simulink model "pid_simulacao"  (R2014a)
settings: Solver=ode3  StartTime=0.0  StopTime=100  FixedStep=0.1  RelTol=1e-3
settings Model: Creator=icaro  LastModifiedBy=Aluno IC

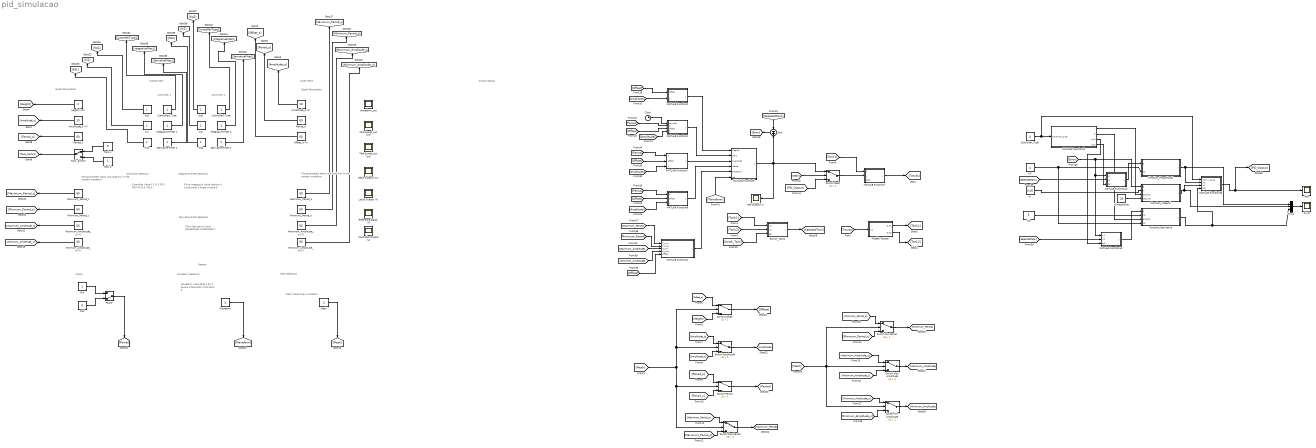
== system pid_simulacao ==
  note: Output Signals
  note: Controller
      | Value
      |
      | P
      | 1
      |
      | PI
      | 2
      |
      | PD
      | 3
      |
      | PID
      | 4
      |
      | PI-D
      | 5
      |
      | I-PD
      | 6
  note: Controller Selection
  note: Signal Parameters
  note: Mesh
      | Value
      |
      | Open
      | 1
      |
      | Closed
      | 2
  note: Mesh Selection
  note: Power
  note: Waveform
      | Value
      |
      | Step
      | 1
      |
      | Sin
      | 2
      |
      | Square
      | 3
      |
      | Sawtooth
      | 4
      |
      | Ramdom
      | 5
  note: Waveform Selection
  note: General
  note: Controller 1
  note: The parameters below are used only in the random waveform
  note: Signal Parameters
  note: The parameters below are used only in the random waveform
  note: Open Mesh
  note: Controller 2
  note: Filtro Derivativo
      | Value
      |
      | Desabilitado
      | 0
      |
      | Habilitado
      | 1
  note: Filtro Integrativo
      | Value
      |
      | Nenhum
      | 0
      |
      | Condicional
      | 1
      |
      | Reset windup
      | 6
  note: Integrative Filter Selection
  note: Derivative Filter Selection
  note: Closed Mesh
  Amplitude_c (V) : Constant  Value=10
  Amplitude_o (V) : Constant  Value=10
  Clock : Clock
  Controller Output (V) : Scope
      settings: TimeRange=10  YMin=2.5  YMax=10  SaveName=meshoutput4
  Controller1 Type : Constant
  Controller2 Type : Constant
  Controller_Type : Constant  Value=4
  Derivative Filter 1 : Constant
  Derivative Filter 2 : Constant
  Function_Derivative : MATLAB Function  TreatAsAtomicUnit=on
  Function_Integral : MATLAB Function  TreatAsAtomicUnit=on
  Function_Proportional : MATLAB Function  TreatAsAtomicUnit=on
  Height (cm) : Constant  Value=2
  Integrative Filter 1 : Constant
  Integrative Filter 2 : Constant
  KD : Constant  Value=5
  KI : Constant  Value=0.05
  KP : Constant  Value=4
  Kd1 : Constant
  Kd2 : Constant
  Ki1 : Constant
  Ki2 : Constant
  Kp1 : Constant
  Kp2 : Constant
  Locks Output (V) : Scope
      settings: TimeRange=10  YMin=2.5  YMax=10  SaveName=meshoutput2
  MATLAB Function1 : MATLAB Function  TreatAsAtomicUnit=on
  MATLAB Function11 : MATLAB Function  TreatAsAtomicUnit=on
  MATLAB Function13 : MATLAB Function  TreatAsAtomicUnit=on
  MATLAB Function14 : MATLAB Function  TreatAsAtomicUnit=on
  MATLAB Function16 : MATLAB Function  TreatAsAtomicUnit=on
  MATLAB Function2 : MATLAB Function  TreatAsAtomicUnit=on
  MATLAB Function3 : MATLAB Function  TreatAsAtomicUnit=on
  MATLAB Function4 : MATLAB Function  TreatAsAtomicUnit=on
  MATLAB Function5 : MATLAB Function  TreatAsAtomicUnit=on
  MATLAB Function6 : MATLAB Function  TreatAsAtomicUnit=on
  MATLAB Function7 : MATLAB Function  TreatAsAtomicUnit=on
  Maximum_Amplitude_c (V) : Constant  Value=60
  Maximum_Amplitude_o (V) : Constant  Value=60
  Maximum_Period_c : Constant  Value=60
  Maximum_Period_o : Constant  Value=60
  Mesh : Constant  Value=2
  Mesh Output (V)1 : Scope
      settings: TimeRange=10  YMin=2.5  YMax=10  SaveName=meshoutput1
  Minimum_Amplitude_c (V) : Constant  Value=60
  Minimum_Amplitude_o (V) : Constant  Value=60
  Minimum_Period_c : Constant  Value=60
  Minimum_Period_o : Constant  Value=60
  Modelo Tanque : Subsystem
  Mux2 : Mux  Inputs=3
  OFF : Constant  Value=0
  ON : Constant
  Offset_o (V) : Constant  Value=60
  P-I-D : Scope
      settings: ShowLegends=on  TimeRange=300  YMin=-100  YMax=100  SaveName=PID
  PID : Scope
      settings: TimeRange=100  YMin=0  YMax=100
  Period_c : Constant  Value=60
  Period_o : Constant  Value=60
  Power : ManualSwitch  CurrentSetting=0
  Ref Output (V) : Scope
      settings: TimeRange=100  SaveName=muxoutput
  Reference Signal (V) : Scope
      settings: TimeRange=10  YMin=2.5  YMax=10  SaveName=meshoutput3
  Sum : Sum  Inputs=-+
  Switch Amplitude : Switch  Criteria=u2 > Threshold  Threshold=1
  Switch Max Amplitude : Switch  Criteria=u2 > Threshold  Threshold=1
  Switch Max Period : Switch  Criteria=u2 > Threshold  Threshold=1
  Switch Mesh : Switch  Criteria=u2 > Threshold  Threshold=1
  Switch Min Amplitude : Switch  Criteria=u2 > Threshold  Threshold=1
  Switch Min Period : Switch  Criteria=u2 > Threshold  Threshold=1
  Switch Offset : Switch  Criteria=u2 > Threshold  Threshold=1
  Switch Period : Switch  Criteria=u2 > Threshold  Threshold=1
  Switch_Tanks : MATLAB Function  TreatAsAtomicUnit=on
  Tank 1 : Constant  Value=0
  Tank 2 : Constant
  Tank1Level_out (cm) : Scope
      settings: TimeRange=10  YMin=4.125  YMax=4.5  SaveName=muxoutput2
  Tank2Level_out (cm) : Scope
      settings: TimeRange=10  YMin=4.125  YMax=4.5  SaveName=muxoutput3
  Tank_Switch : ManualSwitch
  Waveform : Constant  Value=3
  Waveform_out : Scope
      settings: TimeRange=10  YMin=4.125  YMax=4.5  SaveName=muxoutput1
  WindupValue : Constant  Value=20
  wires:
  Clock/1 -> MATLAB Function1/1(counter)
  MATLAB Function7/1(y) -> [Travas]
  MATLAB Function5/1(y) -> Switch Mesh/1, Ref Output (V)/1, Sum/2
  Switch Mesh/1 -> MATLAB Function7/2(u)
  ON/1 -> Power/1
  OFF/1 -> Power/2
  Tank 1/1 -> Tank_Switch/1
  Tank 2/1 -> Tank_Switch/2
  Function_Proportional/1(y) -> MATLAB Function16/2(pro), Mux2/1
  Function_Integral/1(y) -> MATLAB Function16/3(int), Mux2/2
  Sum/1 -> [Error]
  MATLAB Function11/1(i) -> Function_Integral/3(enable)
  KP/1 -> Function_Derivative/4(Kp), Function_Proportional/2(Kp)
  MATLAB Function11/2(d) -> Function_Derivative/3(enable)
  Controller_Type/1 -> MATLAB Function16/1(control_type), MATLAB Function11/1(controller_type)
  MATLAB Function16/1(y) -> [PID_Output], PID/1
  Mux2/1 -> P-I-D/1
  MATLAB Function13/1(y) -> Function_Derivative/1(e)
  MATLAB Function11/3(swd) -> MATLAB Function13/3(sel)
  MATLAB Function14/1(y) -> Function_Proportional/1(e)
  MATLAB Function11/4(swp) -> MATLAB Function14/3(sel)
  KI/1 -> Function_Integral/2(Ki)
  WindupValue/1 -> Function_Integral/4(sat_max)
  KD/1 -> Function_Derivative/2(Kd)
  Function_Derivative/1(y) -> MATLAB Function16/4(der), Mux2/3
  [Travas] -> Modelo Tanque/1(In1)
  Modelo Tanque/1(Out1) -> [Tank1]
  Modelo Tanque/2(Out2) -> [Tank2]
  [Tank1] -> MATLAB Function7/1(h)
  Height (cm)/1 -> [Height]
  Tank_Switch/1 -> [Tank_Switch]
  Amplitude_c (V)/1 -> [Amplitude_c]
  Period_c/1 -> [Period_c]
  Maximum_Period_c/1 -> [Maximum_Period_c]
  Minimum_Period_c/1 -> [Minimum_Period_c]
  Maximum_Amplitude_c (V)/1 -> [Maximum_Amplitude_c]
  Minimum_Amplitude_c (V)/1 -> [Minimum_Amplitude_c]
  Waveform/1 -> [Waveform]
  Mesh/1 -> [Mesh]
  Power/1 -> [Power]
  Amplitude_o (V)/1 -> [Amplitude_o]
  Period_o/1 -> [Period_o]
  Offset_o (V)/1 -> [Offset_o]
  Maximum_Period_o/1 -> [Maximum_Period_o]
  Minimum_Period_o/1 -> [Minimum_Period_o]
  Maximum_Amplitude_o (V)/1 -> [Maximum_Amplitude_o]
  Minimum_Amplitude_o (V)/1 -> [Minimum_Amplitude_o]
  [Mesh] -> Switch Max Period/2, Switch Period/2, Switch Offset/2, Switch Amplitude/2
  [Height] -> Switch Offset/3
  [Offset_o] -> Switch Offset/1
  [Amplitude_o] -> Switch Amplitude/1
  [Amplitude_c] -> Switch Amplitude/3
  [Period_c] -> Switch Period/3
  [Period_o] -> Switch Period/1
  [Maximum_Period_c] -> Switch Max Period/3
  [Maximum_Period_o] -> Switch Max Period/1
  [Minimum_Period_c] -> Switch Min Period/3
  [Minimum_Period_o] -> Switch Min Period/1
  [Maximum_Amplitude_c] -> Switch Max Amplitude/3
  [Maximum_Amplitude_o] -> Switch Max Amplitude/1
  [Minimum_Amplitude_o] -> Switch Min Amplitude/1
  [Minimum_Amplitude_c] -> Switch Min Amplitude/3
  Switch Offset/1 -> [Offset]
  Switch Amplitude/1 -> [Amplitude]
  Switch Period/1 -> [Period]
  Switch Max Period/1 -> [Maximum_Period]
  Switch Min Period/1 -> [Minimum_Period]
  Switch Min Amplitude/1 -> [Minimum_Amplitude]
  Switch Max Amplitude/1 -> [Maximum_Amplitude]
  [Offset] -> MATLAB Function2/1(offset)
  [Amplitude] -> MATLAB Function2/2(A)
  [Amplitude] -> MATLAB Function1/4(A)
  [Offset] -> MATLAB Function1/3(offset)
  [Period] -> MATLAB Function1/2(T)
  [Amplitude] -> MATLAB Function6/3(A)
  [Offset] -> MATLAB Function6/2(offset)
  [Period] -> MATLAB Function6/1(T)
  [SelectedTank] -> MATLAB Function13/2(x2)
  [SelectedTank] -> MATLAB Function14/2(x2)
  [Tank2] -> Switch_Tanks/2(x2)
  [Tank1] -> Switch_Tanks/1(x1)
  Switch_Tanks/1(y) -> [SelectedTank]
  [Switch_Tank] -> Switch_Tanks/3(sel)
  [Offset] -> MATLAB Function3/2(offset)
  [Period] -> MATLAB Function3/1(T)
  [Amplitude] -> MATLAB Function3/3(A)
  [Maximum_Period] -> MATLAB Function4/1(T_min)
  [Minimum_Period] -> MATLAB Function4/2(T_max)
  [Maximum_Amplitude] -> MATLAB Function4/3(A_min)
  [Minimum_Amplitude] -> MATLAB Function4/4(A_max)
  [Offset] -> MATLAB Function4/5(offset)
  MATLAB Function4/1(y) -> MATLAB Function5/5(aleatoria)
  [Waveform] -> MATLAB Function5/6(sel)
  MATLAB Function6/1(y) -> MATLAB Function5/4(dente)
  MATLAB Function3/1(y) -> MATLAB Function5/3(quadrada)
  MATLAB Function1/1(y) -> MATLAB Function5/2(seno)
  MATLAB Function2/1(y) -> MATLAB Function5/1(degrau)
  [Error] -> MATLAB Function14/1(x1), MATLAB Function13/1(x1), Function_Integral/1(e)
  [SelectedTank] -> Sum/1
  [PID_Output] -> Switch Mesh/3
  [Mesh] -> Switch Mesh/2
  [Mesh] -> Switch Min Amplitude/2, Switch Max Amplitude/2, Switch Min Period/2
  Kp1/1 -> [Kp1]
  Ki1/1 -> [Ki1]
  Kd1/1 -> [Kd1]
  Controller1 Type/1 -> [ControllerType1]
  Integrative Filter 1/1 -> [IntegrativeFilter1]
  Derivative Filter 1/1 -> [DerivativeFilter1]
  Kp2/1 -> [Kp2]
  Ki2/1 -> [Ki2]
  Kd2/1 -> [Kd2]
  Derivative Filter 2/1 -> [DerivativeFilter2]
  Integrative Filter 2/1 -> [IntegrativeFilter2]
  Controller2 Type/1 -> [ControllerType2]

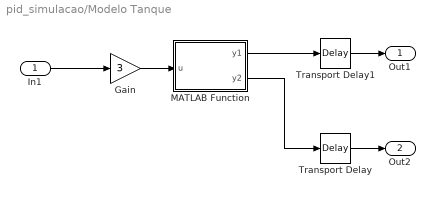
== system pid_simulacao/Modelo Tanque ==
  In1 : Inport
  Gain : Gain  Gain=3
  MATLAB Function : MATLAB Function  TreatAsAtomicUnit=on
  Transport Delay : TransportDelay  DelayTime=2
  Transport Delay1 : TransportDelay  DelayTime=2
  Out1 : Outport
  Out2 : Outport  Port=2
  wires:
  Gain/1 -> MATLAB Function/1(u)
  Transport Delay/1 -> Out2/1
  Transport Delay1/1 -> Out1/1
  MATLAB Function/1(y1) -> Transport Delay1/1
  MATLAB Function/2(y2) -> Transport Delay/1
  In1/1 -> Gain/1

== matlab function pid_simulacao/Modelo Tanque/MATLAB Function ==
  data: u input; y1 output; y2 output
function [y1, y2]= fcn(u)

persistent A1
persistent A2
persistent a1
persistent a2
persistent km
persistent g
persistent t
persistent h1
persistent h2

if(isempty(t))
    A1 = pi*(4.445/2)^2;           %Area transversal do tanque 1
    A2 = pi*(4.445/2)^2;           %Area transversal do tanque 2
    a1 = (0.445/2)^2*pi;     %Area transversal da tubulação de saida em t1 
    a2 =(0.445/2)^2*pi;    %Area transversal da tubulação de saida em t2
    km = 3.3;                %Constante do Motor
    g  = 980.665;               %Constante da gravidade
    h1 = 0;
    h2 = 0;
    t = 10^-1;
end

dh1 = ((km*u) - a1*sqrt(2*g*h1))/A1;
h1 = h1 + t*dh1;
if(h1<0)
    h1 = 0;
end
dh2 = (a1*sqrt(2*g*h1) - a2*sqrt(2*g*h2))/A2;
h2 = h2 + t*dh2;
if(h2<0)
    h2 = 0;
end

y1 = h1;
y2 = h2;

end

== matlab function pid_simulacao/MATLAB Function1 ==
  data: counter input; y output; T input; offset input; A input
function y = seno(counter, T, offset, A)

%counter = cast(counter, 'double');

y = A*sin(counter*2*pi/T) + offset;

== matlab function pid_simulacao/MATLAB Function2 ==
  data: offset input; y output; A input
function y = degrau(offset, A)



y = A + offset;

== matlab function pid_simulacao/MATLAB Function3 ==
  data: y output; T input; offset input; A input
function y = quadrada(T, offset, A)

persistent counter_q;

if isempty(counter_q)
   counter_q = 0; 
end

counter_q = counter_q + 1;

if (counter_q <= 5*T)
    y = -A + offset;
elseif (counter_q > 5*T)
    y = A + offset;
else
    y = 0;
end

if (counter_q >= 10*T)
   counter_q = 0; 
end

== matlab function pid_simulacao/MATLAB Function4 ==
  data: T_min input; y output; T_max input; A_min input; A_max input; offset input
function y = aleatoria(T_min, T_max, A_min, A_max, offset)

persistent T_now;
persistent A_now;
persistent counter_a;

if isempty(counter_a)
    T_now = T_min + (T_max - T_min)*rand;
    A_now = A_min + (A_max - A_min)*rand + offset;
    counter_a = 0;
end

counter_a = counter_a + 1;

y = A_now;

if (counter_a >= T_now*10)
    T_now = T_min + (T_max - T_min)*rand;
    A_now = A_min + (A_max - A_min)*rand + offset;
    counter_a = 0;
end

== matlab function pid_simulacao/MATLAB Function5 ==
  data: degrau input; y output; seno input; quadrada input; dente input; aleatoria input; sel input
function y = mux(degrau, seno, quadrada, dente, aleatoria, sel)

switch sel
    case 1
        y = degrau;
    case 2
        y = seno;
    case 3
        y = quadrada;
    case 4
        y = dente;
    case 5
        y = aleatoria;
    otherwise
        y = 0;
end

== matlab function pid_simulacao/MATLAB Function6 ==
  data: y output; T input; offset input; A input
function y = dente(T, offset, A)

persistent counter_d;

if isempty(counter_d)
   counter_d = 0; 
end


y = counter_d*A*2/(10*T) + offset - A;

counter_d = counter_d + 1;

if (counter_d > T*10)
   counter_d = 0;
end

== matlab function pid_simulacao/Function_Proportional ==
  data: e input; y output; Kp input
function y = proportional(e, Kp)

y = Kp*e;

== matlab function pid_simulacao/MATLAB Function7 ==
  data: h input; u input; y output; start input
    function y = travas(h, u, start)
%#codegen
h_max = 30;

%Trava de tensÃ£o
if(u < -4)
    u = -4;
end
if(u > 4)
    u = 4;
end

%Trava pra nÃ£o sugar ar
if(u < 0 & h < 2)
    u = 0;
end

%Trava de transbordamento
% if(h >= h_max - 1.0 & h < h_max - 0.75)
%    u = 0.95*u;
% elseif(h >= h_max - 0.75 & h < h_max - 0.5)
%     u = 0.93*u;
% elseif(h >= h_max - 0.5 & h < h_max - 0.25)
%     u = 0.91*u;
% elseif(h >= h_max - 0.25 & h < h_max)
%     u = 0.88*u;
% elseif(h >= h_max)
%     u = 0;
% end

%
if h >= (h_max-1)
    u = (h_max - h)*u;
end

%
% persistent goingup
% 
% if isempty(goingup)
%    goingup = 1; 
% end
% 
% if goingup == 1
%    if h >= 29
%       u = 0;
%       goingup = 0;
%    end
% else
%     if h <= 25
%        goingup = 1; 
%     else
%        u = 0; 
%     end
% end
    
y = start*u;

== matlab function pid_simulacao/Function_Integral ==
  data: e input; y output; Ki input; enable input; sat_max input
function y = integral(e, Ki, enable, sat_max)

persistent sum;

if isempty(sum)
   sum = 0; 
end

aux = sum*enable;

if(aux > sat_max) 
    sum = 0;
else
    sum = sum + Ki*e*0.1;
end
y = sum*enable;

== matlab function pid_simulacao/Function_Derivative ==
  data: e input; y output; Kd input; enable input; Kp input
function y = derivative(e, Kd, enable, Kp)

persistent prev_error;

if isempty(prev_error)
   prev_error = 0; 
end

%1/0.1 == 10
Td = Kd/Kp;


y = Kd*(e - prev_error)*enable/0.1;

prev_error = e;

end

== matlab function pid_simulacao/MATLAB Function11 ==
  data: controller_type input; i output; d output; swd output; swp output
function [i,d,swd,swp]= fcn(controller_type)

if(controller_type == 1)
    i = 0;
    d = 0;
    swd = 0;
    swp = 0;
elseif(controller_type == 2)
    i = 1;
    d = 0;
    swd = 0;
    swp = 0;
elseif(controller_type == 3)
    i = 0;
    d = 1;
    swd = 0;
    swp = 0;
elseif(controller_type == 4)
    i = 1;
    d = 1;
    swd = 0;
    swp = 0;
elseif(controller_type == 5)
    i = 1;
    d = 1;
    swd = 1;
    swp = 0;
elseif(controller_type == 6)
    i = 1;
    d = 1;
    swd = 1;
    swp = 1;
else
    i = 0;
    d = 0;
    swd = 0;
    swp = 0;
end

== matlab function pid_simulacao/MATLAB Function13 ==
  data: x1 input; x2 input; y output; sel input
function y = switch_deriv(x1, x2, sel)

if sel == 0
    y = x1; 
else
    y = x2;
end
    
end

== matlab function pid_simulacao/MATLAB Function14 ==
  data: x1 input; x2 input; y output; sel input
function y = switch_prop(x1, x2, sel)

if sel == 0
    y = x1; 
else
    y = x2;
end
    
end

== matlab function pid_simulacao/MATLAB Function16 ==
  data: control_type input; y output; pro input; int input; der input
function y = adding(control_type, pro, int, der)
%#codegen

if(control_type >= 1 && control_type <= 4)
   y = pro + int + der;
elseif(control_type == 5)
    y = pro + int - der;
else
    y = int - pro - der;
end

== matlab function pid_simulacao/Switch_Tanks ==
  data: x1 input; x2 input; y output; sel input
function y = switch2(x1, x2, sel)

if sel == 0
    y = x1; 
else
    y = x2;
end
    
end
